simulink model "Simulator_weighted_inv"  (R2016a)
settings: Solver=ode45  StartTime=0.0  StopTime=100  RelTol=1e-3
values from neighbouring files (symbols this model uses):
  A_Servo = [0 1 0; 0 0 1 ; -B4/B1 -B3/B1 -B2/B1]    [Parameters.m]
  B_Servo = [0 ; 0 ; B0/B1]    [Parameters.m]
  C_Servo = eye(3)    [Parameters.m]
  delay_Kaltitude = 1    [Parameters.m]
  dLMN = [dLdp  0    0 ... (first row only)    [Parameters.m]
  g = 9.81    [Parameters.m]
  I_Pi = diag([8.450e-5 8.450e-5 4.580e-5])    [Parameters.m]
  In = diag([Ixx Iyy Izz])    [Parameters.m]
  InInv = In\eye(3)    [Parameters.m]
  KaD = 5.4    [Parameters.m]
  KaI = 3.6    [Parameters.m]
  KaN = 38    [Parameters.m]
  KaP = 8.0    (= 8)    [Parameters.m]
  Kba = sqrt(KaD/KaI)    [Parameters.m]
  Kbp = sqrt(Kdp/Kip)    [Parameters.m]
  Kbq = sqrt(Kdq/Kiq)    [Parameters.m]
  Kbr = sqrt(Kdr/Kir)    [Parameters.m]
  Kd_E = Kd_N    (= 0.01)    [Parameters.m]
  Kd_N = 0.01    [Parameters.m]
  Kd_u = Kd_v    (= 0.29)    [Parameters.m]
  Kd_v = 0.290    (= 0.29)    [Parameters.m]
  Kdp = 0.00534    [Parameters.m]
  Kdq = Kdp    (= 0.00534)    [Parameters.m]
  Kdr = 0.0153    [Parameters.m]
  Kinv = wpinv(K,W)    [Parameters.m]
  Kip = 0.697    [Parameters.m]
  Kiq = Kip    (= 0.697)    [Parameters.m]
  Kir = 0.125    [Parameters.m]
  Kp_E = Kp_N    (= 0.15)    [Parameters.m]
  Kp_N = 0.15    [Parameters.m]
  Kp_u = Kp_v    (= 6.3)    [Parameters.m]
  Kp_v = 6.3    [Parameters.m]
  KPD = KRD    (= 0.0584)    [Parameters.m]
  KPP = KRP    (= 1.61)    [Parameters.m]
  Kpp = 0.3    [Parameters.m]
  Kpq = Kpp    (= 0.3)    [Parameters.m]
  Kpr = 0.135    [Parameters.m]
  Kq = Cq*ro*A*R^3    (= 2.88925724261e-07)    [Parameters.m]
  KRD = 0.0584    [Parameters.m]
  KRP = 1.61    [Parameters.m]
  Kt = Ct*ro*A*R^2    (= 2.46191978476e-05)    [Parameters.m]
  m = 1.900    (= 1.9)    [Parameters.m]
  Mb = diag([m m m])    [Parameters.m]
  MbInv = Mb\eye(3)    [Parameters.m]
  N = 1/Tf    (= 100)    [Parameters.m]
  N_tras = 100    [Parameters.m]
  pitchMax = pi/6    (= 0.523598775598)    [Parameters.m]
  rollMax = pi/6    (= 0.523598775598)    [Parameters.m]
  satp = 1.5    [Parameters.m]
  satq = 1.5    [Parameters.m]
  satr = 1    [Parameters.m]
  tau = 0.055257    [Parameters.m]
  tc = 1/fc    (= 0.01)    [Parameters.m]
  x1 = [m q]    [Parameters.m]
  yawRateMax = pi/2    (= 1.57079632679)    [Parameters.m]
undefined symbols (not defined in the file or in its folder): Kp, KPI, KRI, sigbuilder_block
libraries: simulink x10, aerolibutil x10
(part 1 of 2)
settings Model: PauseTimes=2  Creator=Claudio  LastModifiedBy=Claudio
settings SolverCC: MaxConsecutiveMinStep=15
settings DataIOCC: SaveFormat=Array
settings HardwareCC: ProdBitPerPointer=32  ProdLargestAtomicFloat=None  ProdIntDivRoundTo=Undefined  ProdEndianess=Unspecified  ProdWordSize=32  ProdHWDeviceType=32-bit Generic
settings ModelReferenceCC: PropagateSignalLabelsOutOfModel=off
settings ConfigComp: CovModelRefEnable=Off

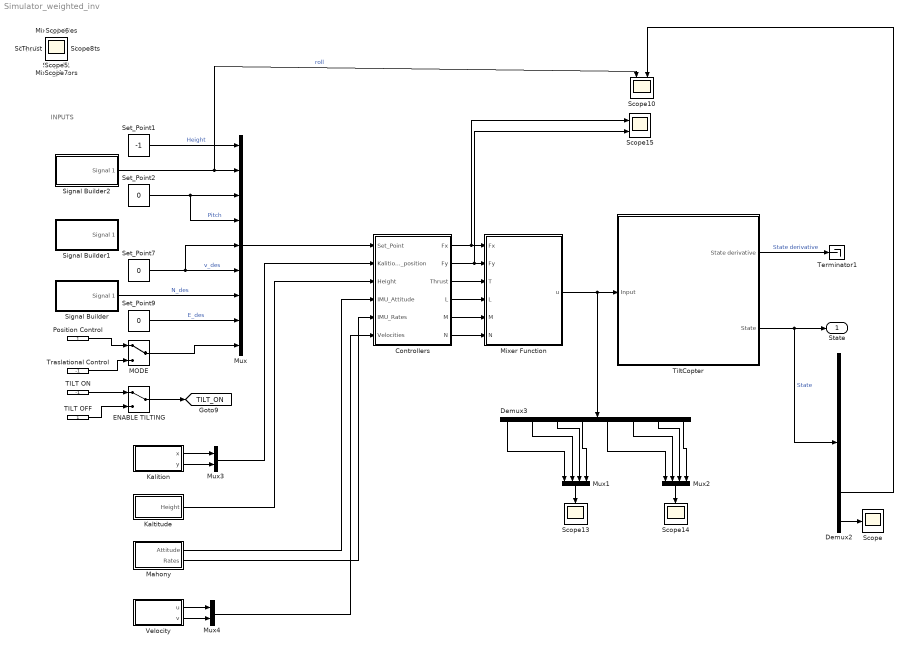
== system Simulator_weighted_inv ==
  note: INPUTS
  Controllers : Subsystem
  Demux2 : Demux  Outputs=12
  Demux3 : Demux  Outputs=8
  ENABLE TILTING : ManualSwitch
  Kalition : Subsystem
  Kaltitude : Subsystem
  MODE : ManualSwitch
  Mahony : Subsystem
  Mixer Function : Subsystem
  Mux : Mux  Inputs=9
  Mux1 : Mux
  Mux2 : Mux
  Mux3 : Mux  Inputs=2
  Mux4 : Mux  Inputs=2
  Position Control : Constant
  Scope{,1..8,11..14} (13 alike) : Scope
  Scope10 : Scope  NumInputPorts=2
  Scope15 : Scope  NumInputPorts=2
  Set_Point1 : Constant  Value=-1
  Set_Point2 : Constant  Value=0
  Set_Point7 : Constant  Value=0
  Set_Point9 : Constant  Value=0
  Signal Builder : Subsystem  Tag=STV Subsys  LoadFcn=sigbuilder_block('load');  StartFcn=sigbuilder_block('start');  StopFcn=sigbuilder_block('stop');  ClipboardFcn=sigbuilder_block('clipboard');  mask(Sigbuilder block){}
      mask help: Simulink:masks:SigbuilderBlock_MD
      mask init:
      | if ~strcmp(get_param(bdroot(gcbh),'SimulationStatus'),'stopped') tuvar = sigbuilder_block('maskInit'); end
      settings: CopyFcn=sigbuilder_block('copy');  DeleteFcn=sigbuilder_block('delete');  ModelCloseFcn=sigbuilder_block('modelClose');  PreSaveFcn=sigbuilder_block('preSave');  PauseFcn=sigbuilder_block('pause');  ContinueFcn=sigbuilder_block('continue');  NameChangeFcn=sigbuilder_block('namechange');  OpenFcn=sigbuilder_block('open',[240 98.25 550.5 359.25 ]);  CloseFcn=sigbuilder_block('close');
      mask Display: plot(0, 0, 100, 100,[2, 2, 32, 32, 2], [68, 8, 8, 68, 68],[32, 2], [38, 38], [32, 19, 2],[53, 60, 44], [32, 17, 17, 2],[16, 16, 31, 31]);txt = getActiveGroup(gcbh);text(2, 100, txt,'verticalAlignment', 'top');
  Signal Builder1 : Subsystem  Tag=STV Subsys  LoadFcn=sigbuilder_block('load');  StartFcn=sigbuilder_block('start');  StopFcn=sigbuilder_block('stop');  ClipboardFcn=sigbuilder_block('clipboard');  mask(Sigbuilder block){}
      mask help: Simulink:masks:SigbuilderBlock_MD
      mask init:
      | if ~strcmp(get_param(bdroot(gcbh),'SimulationStatus'),'stopped') tuvar = sigbuilder_block('maskInit'); end
      settings: CopyFcn=sigbuilder_block('copy');  DeleteFcn=sigbuilder_block('delete');  ModelCloseFcn=sigbuilder_block('modelClose');  PreSaveFcn=sigbuilder_block('preSave');  PauseFcn=sigbuilder_block('pause');  ContinueFcn=sigbuilder_block('continue');  NameChangeFcn=sigbuilder_block('namechange');  OpenFcn=sigbuilder_block('open',[437.25 153 550.5 359.25 ]);  CloseFcn=sigbuilder_block('close');
      mask Display: plot(0, 0, 100, 100,[2, 2, 32, 32, 2], [68, 8, 8, 68, 68],[32, 2], [38, 38], [32, 19, 2],[53, 60, 44], [32, 17, 17, 2],[16, 16, 31, 31]);txt = getActiveGroup(gcbh);text(2, 100, txt,'verticalAlignment', 'top');
  Signal Builder2 : Subsystem  Tag=STV Subsys  LoadFcn=sigbuilder_block('load');  StartFcn=sigbuilder_block('start');  StopFcn=sigbuilder_block('stop');  ClipboardFcn=sigbuilder_block('clipboard');  mask(Sigbuilder block){}
      mask help: Simulink:masks:SigbuilderBlock_MD
      mask init:
      | if ~strcmp(get_param(bdroot(gcbh),'SimulationStatus'),'stopped') tuvar = sigbuilder_block('maskInit'); end
      settings: CopyFcn=sigbuilder_block('copy');  DeleteFcn=sigbuilder_block('delete');  ModelCloseFcn=sigbuilder_block('modelClose');  PreSaveFcn=sigbuilder_block('preSave');  PauseFcn=sigbuilder_block('pause');  ContinueFcn=sigbuilder_block('continue');  NameChangeFcn=sigbuilder_block('namechange');  OpenFcn=sigbuilder_block('open',[437.25 153 550.5 359.25 ]);  CloseFcn=sigbuilder_block('close');
      mask Display: plot(0, 0, 100, 100,[2, 2, 32, 32, 2], [68, 8, 8, 68, 68],[32, 2], [38, 38], [32, 19, 2],[53, 60, 44], [32, 17, 17, 2],[16, 16, 31, 31]);txt = getActiveGroup(gcbh);text(2, 100, txt,'verticalAlignment', 'top');
  TILT OFF : Constant
  TILT ON : Constant  Value=-1
  Terminator1 : Terminator
  TiltCopter : Subsystem
      mask Display:
      | image(imread('TiltCopter_Model.png'))
      | port_label('input',1,'u')
      | port_label('output',1,'Xdot')
      | port_label('output',2,'X')
  Traslational Control : Constant  Value=-1
  Velocity : Subsystem
  State : Outport
  Forces : Scope
  Mixer_Angles : Scope
  Mixer_Motors : Scope
  Moments : Scope
  Thrust : Scope
  tag scope: TILT_ON=global
  wires:
  TiltCopter/2(State) -> Demux2/1, State/1  "State"
  TiltCopter/1(State derivative) -> Terminator1/1  "State derivative"
  Controllers/3(Thrust) -> Mixer Function/3(T)
  Controllers/4(L) -> Mixer Function/4(L)
  Controllers/5(M) -> Mixer Function/5(M)
  Set_Point1/1 -> Mux/1  "Height"
  Set_Point2/1 -> Mux/4, Mux/3  "Pitch"
  Mux/1 -> Controllers/1(Set_Point)
  Set_Point7/1 -> Mux/5, Mux/6  "v_des"
  Set_Point9/1 -> Mux/8  "E_des"
  Position Control/1 -> MODE/1
  Traslational Control/1 -> MODE/2
  MODE/1 -> Mux/9
  Mixer Function/1(u) -> Demux3/1, TiltCopter/1(Input)
  Mux1/1 -> Scope13/1
  Demux3/1 -> Mux1/1
  Demux3/2 -> Mux1/2
  Demux3/3 -> Mux1/3
  Demux3/4 -> Mux1/4
  Mux2/1 -> Scope14/1
  Demux3/5 -> Mux2/1
  Demux3/6 -> Mux2/2
  Demux3/7 -> Mux2/3
  Demux3/8 -> Mux2/4
  Kalition/2(y) -> Mux3/2
  Kalition/1(x) -> Mux3/1
  Mux3/1 -> Controllers/2(Kalition_position)
  Kaltitude/1(Height) -> Controllers/3(Height)
  Mahony/1(Attitude) -> Controllers/4(IMU_Attitude)
  Mahony/2(Rates) -> Controllers/5(IMU_Rates)
  Velocity/2(v) -> Mux4/2
  Velocity/1(u) -> Mux4/1
  Mux4/1 -> Controllers/6(Velocities)
  Controllers/1(Fx) -> Scope15/1, Mixer Function/1(Fx)
  Controllers/2(Fy) -> Scope15/2, Mixer Function/2(Fy)
  TILT ON/1 -> ENABLE TILTING/1
  TILT OFF/1 -> ENABLE TILTING/2
  ENABLE TILTING/1 -> [TILT_ON]
  Controllers/6(N) -> Mixer Function/6(N)
  Signal Builder2/1(Signal 1) -> Scope10/1, Mux/2  "roll"
  Demux2/10 -> Scope10/2
  Demux2/12 -> Scope/1
  Signal Builder/1(Signal 1) -> Mux/7  "N_des"

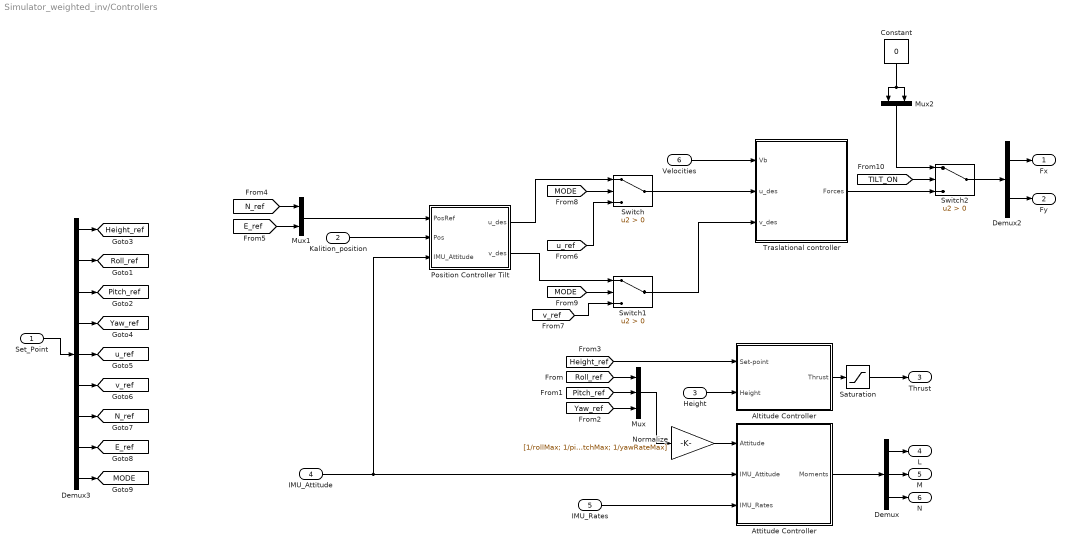
== system Simulator_weighted_inv/Controllers ==
  Set_Point : Inport
  Kalition_position : Inport  Port=2
  Height : Inport  Port=3
  IMU_Attitude : Inport  Port=4
  IMU_Rates : Inport  Port=5
  Velocities : Inport  Port=6
  Altitude Controller : Subsystem
  Attitude Controller : Subsystem
  Constant : Constant  Value=0
  Demux : Demux  Outputs=3
  Demux2 : Demux  Outputs=2
  Demux3 : Demux  Outputs=9
  Mux : Mux  Inputs=3
  Mux1 : Mux  Inputs=2
  Mux2 : Mux  Inputs=2
  Normalize : Gain  Gain=[1/rollMax; 1/pitchMax; 1/yawRateMax]
  Position Controller Tilt : Subsystem
  Saturation : Saturate  UpperLimit=0  LowerLimit=-80
  Switch : Switch  Criteria=u2 > Threshold
  Switch1 : Switch  Criteria=u2 > Threshold
  Switch2 : Switch  Criteria=u2 > Threshold
  Traslational controller : Subsystem
  Fx : Outport
  Fy : Outport  Port=2
  Thrust : Outport  Port=3
  L : Outport  Port=4
  M : Outport  Port=5
  N : Outport  Port=6
  tag scope: E_ref=global, Height_ref=global, MODE=global, N_ref=global, Pitch_ref=global, Roll_ref=global, Yaw_ref=global, u_ref=global, v_ref=global
  wires:
  IMU_Rates/1 -> Attitude Controller/3(IMU_Rates)
  Demux/1 -> L/1
  Demux/2 -> M/1
  Demux/3 -> N/1
  [Pitch_ref] -> Mux/2
  [Yaw_ref] -> Mux/3
  IMU_Attitude/1 -> Position Controller Tilt/3(IMU_Attitude), Attitude Controller/2(IMU_Attitude)
  Mux/1 -> Normalize/1
  Normalize/1 -> Attitude Controller/1(Attitude)
  [Height_ref] -> Altitude Controller/1(Set-point)
  Height/1 -> Altitude Controller/2(Height)
  Altitude Controller/1(Thrust) -> Saturation/1
  Saturation/1 -> Thrust/1
  Attitude Controller/1(Moments) -> Demux/1
  [Roll_ref] -> Mux/1
  Demux2/1 -> Fx/1
  Demux2/2 -> Fy/1
  Velocities/1 -> Traslational controller/1(Vb)
  Set_Point/1 -> Demux3/1
  Demux3/2 -> [Roll_ref]
  Demux3/1 -> [Height_ref]
  Demux3/3 -> [Pitch_ref]
  Demux3/4 -> [Yaw_ref]
  Demux3/5 -> [u_ref]
  Demux3/6 -> [v_ref]
  Demux3/7 -> [N_ref]
  Demux3/8 -> [E_ref]
  Mux1/1 -> Position Controller Tilt/1(PosRef)
  Kalition_position/1 -> Position Controller Tilt/2(Pos)
  [N_ref] -> Mux1/1
  [E_ref] -> Mux1/2
  Demux3/9 -> [MODE]
  Position Controller Tilt/1(u_des) -> Switch/1
  Position Controller Tilt/2(v_des) -> Switch1/1
  Switch/1 -> Traslational controller/2(u_des)
  [u_ref] -> Switch/3
  [v_ref] -> Switch1/3
  [MODE] -> Switch/2
  [MODE] -> Switch1/2
  Switch1/1 -> Traslational controller/3(v_des)
  Switch2/1 -> Demux2/1
  Traslational controller/1(Forces) -> Switch2/3
  Constant/1 -> Mux2/1, Mux2/2
  Mux2/1 -> Switch2/1
  [TILT_ON] -> Switch2/2

== system Simulator_weighted_inv/Kalition ==
  Demux : Demux  Outputs=3
  Terminator : Terminator
  x : Outport
  y : Outport  Port=2
  wires:
  Demux/1 -> x/1  "x"
  Demux/3 -> Terminator/1  "z"
  Demux/2 -> y/1  "y"
  [P_b] -> Demux/1

== system Simulator_weighted_inv/Kaltitude ==
  Bias_u : Bias
  Demux : Demux  Outputs=3
  Sum : Sum  Inputs=|++
  Terminator1 : Terminator
  Terminator2 : Terminator
  Transport Delay : TransportDelay  DelayTime=delay_Kaltitude*tc
  White Noise_u : RandomNumber  DisableCoverage=on  Variance=0*0.00001  SampleTime=0.01
  Zero-Order Hold : ZeroOrderHold  SampleTime=tc
  Height : Outport
  wires:
  Sum/1 -> Zero-Order Hold/1
  Demux/2 -> Terminator1/1  "E"
  [P_e] -> Demux/1
  Bias_u/1 -> Sum/1
  White Noise_u/1 -> Sum/2
  Demux/1 -> Terminator2/1  "N"
  Zero-Order Hold/1 -> Transport Delay/1
  Demux/3 -> Bias_u/1  "D"
  Transport Delay/1 -> Height/1

== system Simulator_weighted_inv/Mahony ==
  Attitude : Outport
  Rates : Outport  Port=2
  wires:
  [Omega_b] -> Rates/1
  [Alpha_e] -> Attitude/1

== system Simulator_weighted_inv/Mixer Function ==
  Fx : Inport
  Fy : Inport  Port=2
  T : Inport  Port=3
  L : Inport  Port=4
  M : Inport  Port=5
  N : Inport  Port=6
  Mux2 : Mux  Inputs=8
  To Workspace : ToWorkspace  VariableName=Uscita_quad  SaveFormat=Structure With Time  SampleTime=-1
  Weighted mixer : Subsystem
  u : Outport
  wires:
  Mux2/1 -> u/1, To Workspace/1
  Fy/1 -> Weighted mixer/2(Fy)
  Fx/1 -> Weighted mixer/1(Fx)
  T/1 -> Weighted mixer/3(T)
  M/1 -> Weighted mixer/5(M)
  Weighted mixer/4(Th4 [%]) -> Mux2/4
  Weighted mixer/3(Th3 [%]) -> Mux2/3
  Weighted mixer/2(Th2 [%]) -> Mux2/2
  Weighted mixer/1(Th1 [%]) -> Mux2/1
  Weighted mixer/5(Alpha1 [deg]) -> Mux2/5
  Weighted mixer/7(Alpha3 [deg]) -> Mux2/7
  Weighted mixer/8(Alpha4 [deg]) -> Mux2/8
  Weighted mixer/6(Alpha2 [deg]) -> Mux2/6
  L/1 -> Weighted mixer/4(L)
  N/1 -> Weighted mixer/6(N)

== system Simulator_weighted_inv/Signal Builder ==
  Demux : Demux  Tag=STV Demux  Outputs=1
  FromWs : FromWorkspace  Tag=STV FromWs  VariableName=tuvar  SampleTime=0
      SigBuilderData=|
      | common.afterFinalStr = 'Extrapolate'
      | common.sampleTime = 0
      | dataSet.timeRange = [0 40]
      | dataSet.name = 'Group 1'
      | sbobj.Groups.Name = 'Group 1'
      | sbobj.Groups.Signals.Name = 'Signal 1'
      | sbobj.Groups.Signals.XData = [0 20 23 40]
      | sbobj.Groups.Signals.YData = [0 0 0.99 1]
      | sbobj.Groups.TimeRange = [0 40]
  Signal 1 : Outport  Tag=STV Outport
  wires:
  Demux/1 -> Signal 1/1
  FromWs/1 -> Demux/1

== system Simulator_weighted_inv/Signal Builder1 ==
  Demux : Demux  Tag=STV Demux  Outputs=1
  FromWs : FromWorkspace  Tag=STV FromWs  VariableName=tuvar  SampleTime=0
      SigBuilderData=|
      | common.afterFinalStr = 'Extrapolate'
      | common.sampleTime = 0
      | dataSet.timeRange = [0 10]
      | dataSet.name = 'Group 1'
      | sbobj.Groups.Name = 'Group 1'
      | sbobj.Groups.Signals.Name = 'Signal 1'
      | sbobj.Groups.Signals.XData = [0 2 3 4 5 6 10]
      | sbobj.Groups.Signals.YData = [0 -0.001 0.5 0.5 0 0 0]
  Signal 1 : Outport  Tag=STV Outport
  wires:
  FromWs/1 -> Demux/1
  Demux/1 -> Signal 1/1

== system Simulator_weighted_inv/Signal Builder2 ==
  Demux : Demux  Tag=STV Demux  Outputs=1
  FromWs : FromWorkspace  Tag=STV FromWs  VariableName=tuvar  SampleTime=0
      SigBuilderData=|
      | common.afterFinalStr = 'Extrapolate'
      | common.sampleTime = 0
      | dataSet.timeRange = [0 10]
      | dataSet.name = 'Group 1'
      | sbobj.Groups.Name = 'Group 1'
      | sbobj.Groups.Signals.Name = 'Signal 1'
      | sbobj.Groups.Signals.XData = [0 3 5 7 8.58 10]
      | sbobj.Groups.Signals.YData = [0 0 0.17 0.17 0 0]
  Signal 1 : Outport  Tag=STV Outport
  wires:
  Demux/1 -> Signal 1/1
  FromWs/1 -> Demux/1

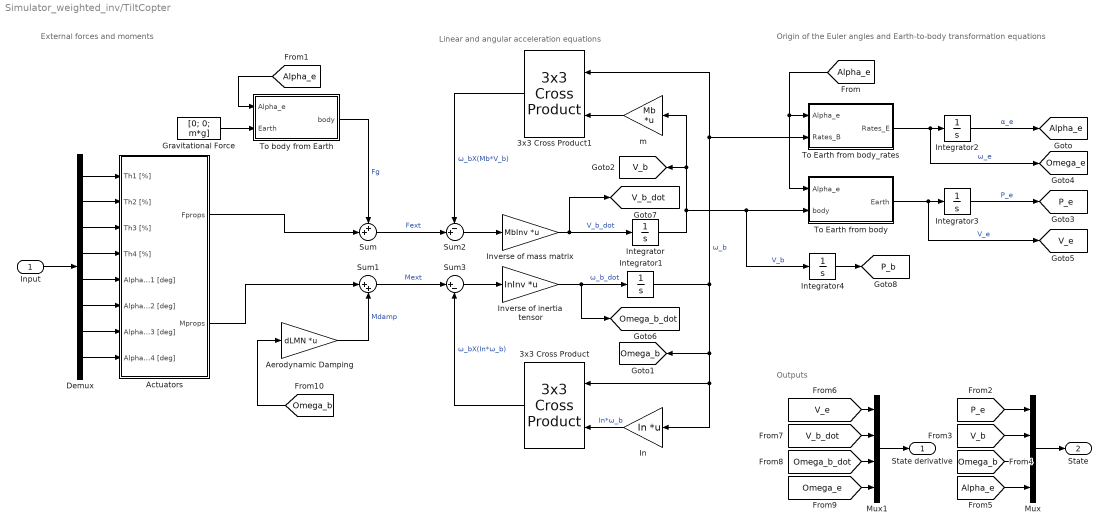
== system Simulator_weighted_inv/TiltCopter ==
  note: External forces and moments
  note: Outputs
  note: Origin of the Euler angles and Earth-to-body transformation equations
  note: Linear and angular acceleration equations
  Input : Inport
  3x3 Cross Product : aerolibutil/3x3 Cross Product
  3x3 Cross Product1 : aerolibutil/3x3 Cross Product
  Actuators : Subsystem
  Aerodynamic Damping : Gain  Gain=dLMN  Multiplication=Matrix(K*u)
  Demux : Demux  Outputs=8
  Gravitational Force : Constant  Value=[0; 0; m*g]
  In : Gain  Gain=In  Multiplication=Matrix(K*u)
  Integrator : Integrator  InitialCondition=[0; 0; 0]  UpperSaturationLimit=20
  Integrator{1..4} (4 alike) : Integrator  InitialCondition=[0; 0; 0]
  Inverse of inertia tensor : Gain  Gain=InInv  Multiplication=Matrix(K*u)
  Inverse of mass matrix : Gain  Gain=MbInv  Multiplication=Matrix(K*u)
  Mux : Mux
  Mux1 : Mux
  Sum : Sum  Inputs=++|
  Sum1 : Sum  Inputs=|++
  Sum2 : Sum  Inputs=-+|
  Sum3 : Sum  Inputs=|+-
  To Earth from body : MATLAB Function  TreatAsAtomicUnit=on
  To Earth from body_rates : MATLAB Function  TreatAsAtomicUnit=on
  To body from Earth : MATLAB Function  TreatAsAtomicUnit=on
  m : Gain  Gain=Mb  Multiplication=Matrix(K*u)
  State derivative : Outport
  State : Outport  Port=2
  tag scope: Alpha_e=global, Omega_b=global, Omega_b_dot=global, Omega_e=global, P_b=global, P_e=global, V_b=global, V_b_dot=global, V_e=global
  wires:
  To Earth from body_rates/1(Rates_E) -> Integrator2/1, [Omega_e]  "ω_e"
  [P_e] -> Mux/1
  3x3 Cross Product/1 -> Sum3/2  "ω_bX(In*ω_b)"
  [V_b_dot] -> Mux1/2
  Mux/1 -> State/1
  Mux1/1 -> State derivative/1
  [V_b] -> Mux/2
  [Alpha_e] -> Mux/4
  [Omega_b] -> Mux/3
  Demux/4 -> Actuators/4(Th4 [%])
  [Omega_e] -> Mux1/4
  [Omega_b_dot] -> Mux1/3
  [V_e] -> Mux1/1
  Demux/3 -> Actuators/3(Th3 [%])
  Inverse of mass matrix/1 -> Integrator/1, [V_b_dot]  "V_b_dot"
  Integrator/1 -> Integrator4/1, To Earth from body/2(body), m/1, [V_b]  "V_b"
  [Alpha_e] -> To Earth from body/1(Alpha_e), To Earth from body_rates/1(Alpha_e)
  Integrator1/1 -> To Earth from body_rates/2(Rates_B), 3x3 Cross Product1/1, 3x3 Cross Product/1, In/1, [Omega_b]  "ω_b"
  Sum3/1 -> Inverse of inertia tensor/1
  Sum2/1 -> Inverse of mass matrix/1
  m/1 -> 3x3 Cross Product1/2
  Sum/1 -> Sum2/2  "Fext"
  Sum1/1 -> Sum3/1  "Mext"
  Demux/1 -> Actuators/1(Th1 [%])
  Demux/2 -> Actuators/2(Th2 [%])
  Inverse of inertia tensor/1 -> Integrator1/1, [Omega_b_dot]  "ω_b_dot"
  3x3 Cross Product1/1 -> Sum2/1  "ω_bX(Mb*V_b)"
  Integrator2/1 -> [Alpha_e]  "α_e"
  Aerodynamic Damping/1 -> Sum1/2  "Mdamp"
  Integrator3/1 -> [P_e]  "P_e"
  In/1 -> 3x3 Cross Product/2  "In*ω_b"
  [Omega_b] -> Aerodynamic Damping/1
  To Earth from body/1(Earth) -> [V_e], Integrator3/1  "V_e"
  To body from Earth/1(body) -> Sum/1  "Fg"
  Gravitational Force/1 -> To body from Earth/2(Earth)
  [Alpha_e] -> To body from Earth/1(Alpha_e)
  Input/1 -> Demux/1
  Demux/5 -> Actuators/5(Alpha_1 [deg])
  Demux/6 -> Actuators/6(Alpha_2 [deg])
  Demux/7 -> Actuators/7(Alpha_3 [deg])
  Demux/8 -> Actuators/8(Alpha_4 [deg])
  Actuators/1(Fprops) -> Sum/2
  Actuators/2(Mprops) -> Sum1/1
  Integrator4/1 -> [P_b]

== system Simulator_weighted_inv/Velocity ==
  Demux : Demux  Outputs=3
  Terminator : Terminator
  u : Outport
  v : Outport  Port=2
  wires:
  Demux/2 -> v/1  "v"
  [V_b] -> Demux/1
  Demux/3 -> Terminator/1  "w"
  Demux/1 -> u/1  "u"

== system Simulator_weighted_inv/Controllers/Altitude Controller ==
  Set-point : Inport
  Height : Inport  Port=2
  Constant : Constant  Value=m*g
  Normalize : Gain
  PD Controller : simulink/Continuous/PID Controller  Controller=PID  TimeDomain=Continuous-time  SampleTime=-1  IntegratorMethod=Forward Euler  FilterMethod=Trapezoidal  Form=Parallel  UseFilter=on  ControllerParametersSource=internal  P=KaP  I=KaI  D=KaD  N=KaN  InitialConditionSource=internal  InitialConditionForIntegrator=0  InitialConditionForFilter=0  ExternalReset=none  LimitOutput=on  UpperSaturationLimit=10  LowerSaturationLimit=-10  LinearizeAsGain=on  AntiWindupMode=back-calculation  Kb=Kba  TrackingMode=off  Kt=1  PParamMin=[]  PParamMax=[]  IParamMin=[]  IParamMax=[]  DParamMin=[]  DParamMax=[]  NParamMin=[]  NParamMax=[]  KbParamMin=[]  KbParamMax=[]  KtParamMin=[]  KtParamMax=[]  POutMin=[]  POutMax=[]  IOutMin=[]  IOutMax=[]  DOutMin=[]  DOutMax=[]  NOutMin=[]  NOutMax=[]  KbOutMin=[]  KbOutMax=[]  KtOutMin=[]  KtOutMax=[]  IntegratorOutMin=[]  IntegratorOutMax=[]  FilterOutMin=[]  FilterOutMax=[]  SumOutMin=[]  SumOutMax=[]  SumI1OutMin=[]  SumI1OutMax=[]  SumI2OutMin=[]  SumI2OutMax=[]  SumI3OutMin=[]  SumI3OutMax=[]  SumDOutMin=[]  SumDOutMax=[]  SaturationOutMin=[]  SaturationOutMax=[]  IntegratorContinuousStateAttributes=''  IntegratorStateMustResolveToSignalObject=off  IntegratorRTWStateStorageClass=Auto  FilterContinuousStateAttributes=''  FilterStateMustResolveToSignalObject=off  FilterRTWStateStorageClass=Auto  DifferentiatorICPrevScaledInput=0  DifferentiatorOutMin=[]  DifferentiatorOutMax=[]
  Sum1 : Sum  Inputs=-+|
  Sum2 : Sum  Inputs=|+-
  Thrust : Outport
  wires:
  Sum2/1 -> PD Controller/1
  Height/1 -> Sum2/2
  Sum1/1 -> Thrust/1
  Constant/1 -> Sum1/1
  Set-point/1 -> Sum2/1
  PD Controller/1 -> Normalize/1
  Normalize/1 -> Sum1/2

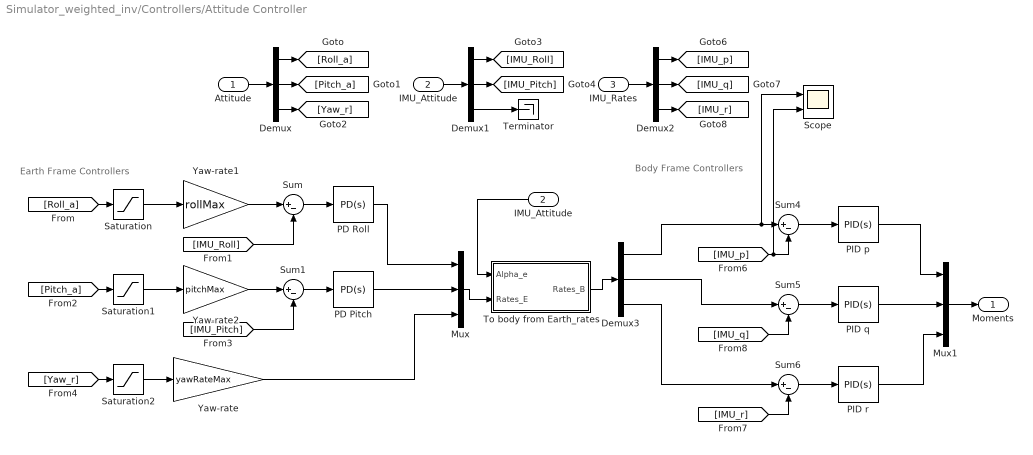
== system Simulator_weighted_inv/Controllers/Attitude Controller ==
  note: Body Frame Controllers
  note: Earth Frame Controllers
  Attitude : Inport
  IMU_Attitude : Inport  Port=2
  IMU_Rates : Inport  Port=3
  Demux{,1..3} (4 alike) : Demux  Outputs=3
  "IMU_Attitude " : InportShadow  Port=2
  Mux : Mux  Inputs=3
  Mux1 : Mux  Inputs=3
  PD Pitch : simulink/Continuous/PID Controller  Controller=PD  TimeDomain=Continuous-time  SampleTime=-1  IntegratorMethod=Forward Euler  FilterMethod=Forward Euler  Form=Parallel  UseFilter=on  ControllerParametersSource=internal  P=KPP  I=KPI  D=KPD  N=N  InitialConditionSource=internal  InitialConditionForIntegrator=0  InitialConditionForFilter=0  ExternalReset=none  LimitOutput=off  UpperSaturationLimit=inf  LowerSaturationLimit=-inf  LinearizeAsGain=on  AntiWindupMode=none  Kb=1  TrackingMode=off  Kt=1  PParamMin=[]  PParamMax=[]  IParamMin=[]  IParamMax=[]  DParamMin=[]  DParamMax=[]  NParamMin=[]  NParamMax=[]  KbParamMin=[]  KbParamMax=[]  KtParamMin=[]  KtParamMax=[]  POutMin=[]  POutMax=[]  IOutMin=[]  IOutMax=[]  DOutMin=[]  DOutMax=[]  NOutMin=[]  NOutMax=[]  KbOutMin=[]  KbOutMax=[]  KtOutMin=[]  KtOutMax=[]  IntegratorOutMin=[]  IntegratorOutMax=[]  FilterOutMin=[]  FilterOutMax=[]  SumOutMin=[]  SumOutMax=[]  SumI1OutMin=[]  SumI1OutMax=[]  SumI2OutMin=[]  SumI2OutMax=[]  SumI3OutMin=[]  SumI3OutMax=[]  SumDOutMin=[]  SumDOutMax=[]  SaturationOutMin=[]  SaturationOutMax=[]  IntegratorContinuousStateAttributes=''  IntegratorStateMustResolveToSignalObject=off  IntegratorRTWStateStorageClass=Auto  FilterContinuousStateAttributes=''  FilterStateMustResolveToSignalObject=off  FilterRTWStateStorageClass=Auto  DifferentiatorICPrevScaledInput=0  DifferentiatorOutMin=[]  DifferentiatorOutMax=[]
  PD Roll : simulink/Continuous/PID Controller  Controller=PD  TimeDomain=Continuous-time  SampleTime=-1  IntegratorMethod=Forward Euler  FilterMethod=Forward Euler  Form=Parallel  UseFilter=on  ControllerParametersSource=internal  P=KRP  I=KRI  D=KRD  N=N  InitialConditionSource=internal  InitialConditionForIntegrator=0  InitialConditionForFilter=0  ExternalReset=none  LimitOutput=off  UpperSaturationLimit=inf  LowerSaturationLimit=-inf  LinearizeAsGain=on  AntiWindupMode=none  Kb=1  TrackingMode=off  Kt=1  PParamMin=[]  PParamMax=[]  IParamMin=[]  IParamMax=[]  DParamMin=[]  DParamMax=[]  NParamMin=[]  NParamMax=[]  KbParamMin=[]  KbParamMax=[]  KtParamMin=[]  KtParamMax=[]  POutMin=[]  POutMax=[]  IOutMin=[]  IOutMax=[]  DOutMin=[]  DOutMax=[]  NOutMin=[]  NOutMax=[]  KbOutMin=[]  KbOutMax=[]  KtOutMin=[]  KtOutMax=[]  IntegratorOutMin=[]  IntegratorOutMax=[]  FilterOutMin=[]  FilterOutMax=[]  SumOutMin=[]  SumOutMax=[]  SumI1OutMin=[]  SumI1OutMax=[]  SumI2OutMin=[]  SumI2OutMax=[]  SumI3OutMin=[]  SumI3OutMax=[]  SumDOutMin=[]  SumDOutMax=[]  SaturationOutMin=[]  SaturationOutMax=[]  IntegratorContinuousStateAttributes=''  IntegratorStateMustResolveToSignalObject=off  IntegratorRTWStateStorageClass=Auto  FilterContinuousStateAttributes=''  FilterStateMustResolveToSignalObject=off  FilterRTWStateStorageClass=Auto  DifferentiatorICPrevScaledInput=0  DifferentiatorOutMin=[]  DifferentiatorOutMax=[]
  PID p : simulink/Continuous/PID Controller  Controller=PID  TimeDomain=Continuous-time  SampleTime=-1  IntegratorMethod=Forward Euler  FilterMethod=Forward Euler  Form=Parallel  UseFilter=on  ControllerParametersSource=internal  P=Kpp  I=Kip  D=Kdp  N=N  InitialConditionSource=internal  InitialConditionForIntegrator=0  InitialConditionForFilter=0  ExternalReset=none  LimitOutput=on  UpperSaturationLimit=satp  LowerSaturationLimit=-satp  LinearizeAsGain=on  AntiWindupMode=back-calculation  Kb=Kbp  TrackingMode=off  Kt=1  PParamMin=[]  PParamMax=[]  IParamMin=[]  IParamMax=[]  DParamMin=[]  DParamMax=[]  NParamMin=[]  NParamMax=[]  KbParamMin=[]  KbParamMax=[]  KtParamMin=[]  KtParamMax=[]  POutMin=[]  POutMax=[]  IOutMin=[]  IOutMax=[]  DOutMin=[]  DOutMax=[]  NOutMin=[]  NOutMax=[]  KbOutMin=[]  KbOutMax=[]  KtOutMin=[]  KtOutMax=[]  IntegratorOutMin=[]  IntegratorOutMax=[]  FilterOutMin=[]  FilterOutMax=[]  SumOutMin=[]  SumOutMax=[]  SumI1OutMin=[]  SumI1OutMax=[]  SumI2OutMin=[]  SumI2OutMax=[]  SumI3OutMin=[]  SumI3OutMax=[]  SumDOutMin=[]  SumDOutMax=[]  SaturationOutMin=[]  SaturationOutMax=[]  IntegratorContinuousStateAttributes=''  IntegratorStateMustResolveToSignalObject=off  IntegratorRTWStateStorageClass=Auto  FilterContinuousStateAttributes=''  FilterStateMustResolveToSignalObject=off  FilterRTWStateStorageClass=Auto  DifferentiatorICPrevScaledInput=0  DifferentiatorOutMin=[]  DifferentiatorOutMax=[]
  PID q : simulink/Continuous/PID Controller  Controller=PID  TimeDomain=Continuous-time  SampleTime=-1  IntegratorMethod=Forward Euler  FilterMethod=Forward Euler  Form=Parallel  UseFilter=on  ControllerParametersSource=internal  P=Kpq  I=Kiq  D=Kdq  N=N  InitialConditionSource=internal  InitialConditionForIntegrator=0  InitialConditionForFilter=0  ExternalReset=none  LimitOutput=on  UpperSaturationLimit=satq  LowerSaturationLimit=-satq  LinearizeAsGain=on  AntiWindupMode=back-calculation  Kb=Kbq  TrackingMode=off  Kt=1  PParamMin=[]  PParamMax=[]  IParamMin=[]  IParamMax=[]  DParamMin=[]  DParamMax=[]  NParamMin=[]  NParamMax=[]  KbParamMin=[]  KbParamMax=[]  KtParamMin=[]  KtParamMax=[]  POutMin=[]  POutMax=[]  IOutMin=[]  IOutMax=[]  DOutMin=[]  DOutMax=[]  NOutMin=[]  NOutMax=[]  KbOutMin=[]  KbOutMax=[]  KtOutMin=[]  KtOutMax=[]  IntegratorOutMin=[]  IntegratorOutMax=[]  FilterOutMin=[]  FilterOutMax=[]  SumOutMin=[]  SumOutMax=[]  SumI1OutMin=[]  SumI1OutMax=[]  SumI2OutMin=[]  SumI2OutMax=[]  SumI3OutMin=[]  SumI3OutMax=[]  SumDOutMin=[]  SumDOutMax=[]  SaturationOutMin=[]  SaturationOutMax=[]  IntegratorContinuousStateAttributes=''  IntegratorStateMustResolveToSignalObject=off  IntegratorRTWStateStorageClass=Auto  FilterContinuousStateAttributes=''  FilterStateMustResolveToSignalObject=off  FilterRTWStateStorageClass=Auto  DifferentiatorICPrevScaledInput=0  DifferentiatorOutMin=[]  DifferentiatorOutMax=[]
  PID r : simulink/Continuous/PID Controller  Controller=PID  TimeDomain=Continuous-time  SampleTime=-1  IntegratorMethod=Forward Euler  FilterMethod=Forward Euler  Form=Parallel  UseFilter=on  ControllerParametersSource=internal  P=Kpr  I=Kir  D=Kdr  N=N  InitialConditionSource=internal  InitialConditionForIntegrator=0  InitialConditionForFilter=0  ExternalReset=none  LimitOutput=on  UpperSaturationLimit=satr  LowerSaturationLimit=-satr  LinearizeAsGain=on  AntiWindupMode=back-calculation  Kb=Kbr  TrackingMode=off  Kt=1  PParamMin=[]  PParamMax=[]  IParamMin=[]  IParamMax=[]  DParamMin=[]  DParamMax=[]  NParamMin=[]  NParamMax=[]  KbParamMin=[]  KbParamMax=[]  KtParamMin=[]  KtParamMax=[]  POutMin=[]  POutMax=[]  IOutMin=[]  IOutMax=[]  DOutMin=[]  DOutMax=[]  NOutMin=[]  NOutMax=[]  KbOutMin=[]  KbOutMax=[]  KtOutMin=[]  KtOutMax=[]  IntegratorOutMin=[]  IntegratorOutMax=[]  FilterOutMin=[]  FilterOutMax=[]  SumOutMin=[]  SumOutMax=[]  SumI1OutMin=[]  SumI1OutMax=[]  SumI2OutMin=[]  SumI2OutMax=[]  SumI3OutMin=[]  SumI3OutMax=[]  SumDOutMin=[]  SumDOutMax=[]  SaturationOutMin=[]  SaturationOutMax=[]  IntegratorContinuousStateAttributes=''  IntegratorStateMustResolveToSignalObject=off  IntegratorRTWStateStorageClass=Auto  FilterContinuousStateAttributes=''  FilterStateMustResolveToSignalObject=off  FilterRTWStateStorageClass=Auto  DifferentiatorICPrevScaledInput=0  DifferentiatorOutMin=[]  DifferentiatorOutMax=[]
  Saturation : Saturate  UpperLimit=1  LowerLimit=-1
  Saturation1 : Saturate  UpperLimit=1  LowerLimit=-1
  Saturation2 : Saturate  UpperLimit=1  LowerLimit=-1
  Scope : Scope  NumInputPorts=2
  Sum{,1,4..6} (5 alike) : Sum  Inputs=|+-
  Terminator : Terminator
  To body from Earth_rates : MATLAB Function  TreatAsAtomicUnit=on
  Yaw-rate : Gain  Gain=yawRateMax
  Yaw-rate1 : Gain  Gain=rollMax
  Yaw-rate2 : Gain  Gain=pitchMax
  Moments : Outport
  wires:
  Sum4/1 -> PID p/1
  IMU_Attitude/1 -> Demux1/1
  Attitude/1 -> Demux/1
  Demux/3 -> [Yaw_r]
  IMU_Rates/1 -> Demux2/1
  [IMU_Pitch] -> Sum1/2
  [Pitch_a] -> Saturation1/1
  [IMU_Roll] -> Sum/2
  [Roll_a] -> Saturation/1
  Mux1/1 -> Moments/1
  PD Roll/1 -> Mux/1
  [Yaw_r] -> Saturation2/1
  PD Pitch/1 -> Mux/2
  Sum5/1 -> PID q/1
  PID r/1 -> Mux1/3
  PID p/1 -> Mux1/1
  Sum6/1 -> PID r/1
  PID q/1 -> Mux1/2
  Demux/2 -> [Pitch_a]
  Demux2/3 -> [IMU_r]
  Demux1/1 -> [IMU_Roll]
  Demux/1 -> [Roll_a]
  Demux2/1 -> [IMU_p]
  Demux1/3 -> Terminator/1
  Demux2/2 -> [IMU_q]
  Demux1/2 -> [IMU_Pitch]
  Sum/1 -> PD Roll/1
  Sum1/1 -> PD Pitch/1
  Saturation1/1 -> Yaw-rate2/1
  Yaw-rate1/1 -> Sum/1
  Yaw-rate2/1 -> Sum1/1
  [IMU_p] -> Sum4/2, Scope/2
  Demux3/2 -> Sum5/1
  Demux3/3 -> Sum6/1
  [IMU_q] -> Sum5/2
  [IMU_r] -> Sum6/2
  Yaw-rate/1 -> Mux/3
  Saturation/1 -> Yaw-rate1/1
  Saturation2/1 -> Yaw-rate/1
  "IMU_Attitude "/1 -> To body from Earth_rates/1(Alpha_e)
  Mux/1 -> To body from Earth_rates/2(Rates_E)
  To body from Earth_rates/1(Rates_B) -> Demux3/1
  Demux3/1 -> Scope/1, Sum4/1

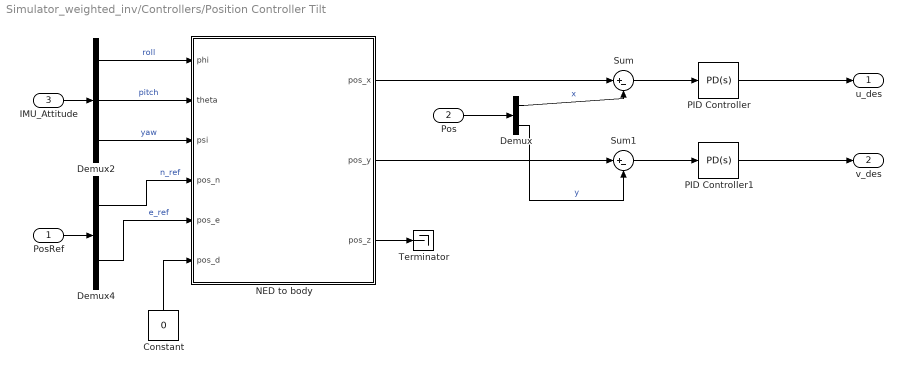
== system Simulator_weighted_inv/Controllers/Position Controller Tilt ==
  PosRef : Inport
  Pos : Inport  Port=2
  IMU_Attitude : Inport  Port=3
  Constant : Constant  Value=0
  Demux : Demux  Outputs=2
  Demux2 : Demux  Outputs=3
  Demux4 : Demux  Outputs=2
  NED to body : MATLAB Function  TreatAsAtomicUnit=on
  PID Controller : simulink/Continuous/PID Controller  Controller=PD  TimeDomain=Continuous-time  SampleTime=-1  IntegratorMethod=Forward Euler  FilterMethod=Forward Euler  Form=Parallel  UseFilter=on  ControllerParametersSource=internal  P=Kp_N  I=1  D=Kd_N  N=100  InitialConditionSource=internal  InitialConditionForIntegrator=0  InitialConditionForFilter=0  ExternalReset=none  LimitOutput=off  UpperSaturationLimit=inf  LowerSaturationLimit=-inf  LinearizeAsGain=on  AntiWindupMode=none  Kb=1  TrackingMode=off  Kt=1  PParamMin=[]  PParamMax=[]  IParamMin=[]  IParamMax=[]  DParamMin=[]  DParamMax=[]  NParamMin=[]  NParamMax=[]  KbParamMin=[]  KbParamMax=[]  KtParamMin=[]  KtParamMax=[]  POutMin=[]  POutMax=[]  IOutMin=[]  IOutMax=[]  DOutMin=[]  DOutMax=[]  NOutMin=[]  NOutMax=[]  KbOutMin=[]  KbOutMax=[]  KtOutMin=[]  KtOutMax=[]  IntegratorOutMin=[]  IntegratorOutMax=[]  FilterOutMin=[]  FilterOutMax=[]  SumOutMin=[]  SumOutMax=[]  SumI1OutMin=[]  SumI1OutMax=[]  SumI2OutMin=[]  SumI2OutMax=[]  SumI3OutMin=[]  SumI3OutMax=[]  SumDOutMin=[]  SumDOutMax=[]  SaturationOutMin=[]  SaturationOutMax=[]  IntegratorContinuousStateAttributes=''  IntegratorStateMustResolveToSignalObject=off  IntegratorRTWStateStorageClass=Auto  FilterContinuousStateAttributes=''  FilterStateMustResolveToSignalObject=off  FilterRTWStateStorageClass=Auto  DifferentiatorICPrevScaledInput=0  DifferentiatorOutMin=[]  DifferentiatorOutMax=[]
  PID Controller1 : simulink/Continuous/PID Controller  Controller=PD  TimeDomain=Continuous-time  SampleTime=-1  IntegratorMethod=Forward Euler  FilterMethod=Forward Euler  Form=Parallel  UseFilter=on  ControllerParametersSource=internal  P=Kp_E  I=1  D=Kd_E  N=100  InitialConditionSource=internal  InitialConditionForIntegrator=0  InitialConditionForFilter=0  ExternalReset=none  LimitOutput=off  UpperSaturationLimit=inf  LowerSaturationLimit=-inf  LinearizeAsGain=on  AntiWindupMode=none  Kb=1  TrackingMode=off  Kt=1  PParamMin=[]  PParamMax=[]  IParamMin=[]  IParamMax=[]  DParamMin=[]  DParamMax=[]  NParamMin=[]  NParamMax=[]  KbParamMin=[]  KbParamMax=[]  KtParamMin=[]  KtParamMax=[]  POutMin=[]  POutMax=[]  IOutMin=[]  IOutMax=[]  DOutMin=[]  DOutMax=[]  NOutMin=[]  NOutMax=[]  KbOutMin=[]  KbOutMax=[]  KtOutMin=[]  KtOutMax=[]  IntegratorOutMin=[]  IntegratorOutMax=[]  FilterOutMin=[]  FilterOutMax=[]  SumOutMin=[]  SumOutMax=[]  SumI1OutMin=[]  SumI1OutMax=[]  SumI2OutMin=[]  SumI2OutMax=[]  SumI3OutMin=[]  SumI3OutMax=[]  SumDOutMin=[]  SumDOutMax=[]  SaturationOutMin=[]  SaturationOutMax=[]  IntegratorContinuousStateAttributes=''  IntegratorStateMustResolveToSignalObject=off  IntegratorRTWStateStorageClass=Auto  FilterContinuousStateAttributes=''  FilterStateMustResolveToSignalObject=off  FilterRTWStateStorageClass=Auto  DifferentiatorICPrevScaledInput=0  DifferentiatorOutMin=[]  DifferentiatorOutMax=[]
  Sum : Sum  Inputs=|+-
  Sum1 : Sum  Inputs=|+-
  Terminator : Terminator
  u_des : Outport
  v_des : Outport  Port=2
  wires:
  Demux4/1 -> NED to body/4(pos_n)  "n_ref"
  Demux4/2 -> NED to body/5(pos_e)  "e_ref"
  PosRef/1 -> Demux4/1
  NED to body/3(pos_z) -> Terminator/1
  IMU_Attitude/1 -> Demux2/1
  Demux2/2 -> NED to body/2(theta)  "pitch"
  Constant/1 -> NED to body/6(pos_d)
  Pos/1 -> Demux/1
  Demux2/3 -> NED to body/3(psi)  "yaw"
  Demux2/1 -> NED to body/1(phi)  "roll"
  Sum/1 -> PID Controller/1
  NED to body/1(pos_x) -> Sum/1
  Demux/1 -> Sum/2  "x"
  PID Controller/1 -> u_des/1
  Sum1/1 -> PID Controller1/1
  NED to body/2(pos_y) -> Sum1/1
  Demux/2 -> Sum1/2  "y"
  PID Controller1/1 -> v_des/1

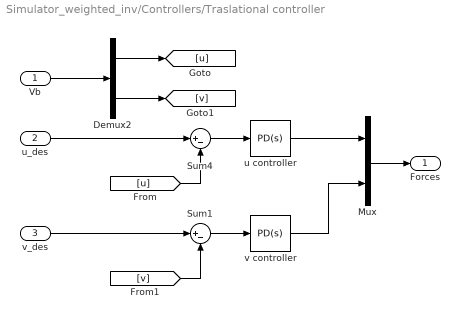
== system Simulator_weighted_inv/Controllers/Traslational controller ==
  Vb : Inport
  u_des : Inport  Port=2
  v_des : Inport  Port=3
  Demux2 : Demux  Outputs=2
  Mux : Mux  Inputs=2
  Sum1 : Sum  Inputs=|+-
  Sum4 : Sum  Inputs=|+-
  u controller : simulink/Continuous/PID Controller  Controller=PD  TimeDomain=Continuous-time  SampleTime=-1  IntegratorMethod=Forward Euler  FilterMethod=Forward Euler  Form=Parallel  UseFilter=on  ControllerParametersSource=internal  P=Kp_u  I=6  D=Kd_u  N=N_tras  InitialConditionSource=internal  InitialConditionForIntegrator=0  InitialConditionForFilter=0  ExternalReset=none  LimitOutput=off  UpperSaturationLimit=inf  LowerSaturationLimit=-inf  LinearizeAsGain=on  AntiWindupMode=none  Kb=1  TrackingMode=off  Kt=1  PParamMin=[]  PParamMax=[]  IParamMin=[]  IParamMax=[]  DParamMin=[]  DParamMax=[]  NParamMin=[]  NParamMax=[]  KbParamMin=[]  KbParamMax=[]  KtParamMin=[]  KtParamMax=[]  POutMin=[]  POutMax=[]  IOutMin=[]  IOutMax=[]  DOutMin=[]  DOutMax=[]  NOutMin=[]  NOutMax=[]  KbOutMin=[]  KbOutMax=[]  KtOutMin=[]  KtOutMax=[]  IntegratorOutMin=[]  IntegratorOutMax=[]  FilterOutMin=[]  FilterOutMax=[]  SumOutMin=[]  SumOutMax=[]  SumI1OutMin=[]  SumI1OutMax=[]  SumI2OutMin=[]  SumI2OutMax=[]  SumI3OutMin=[]  SumI3OutMax=[]  SumDOutMin=[]  SumDOutMax=[]  SaturationOutMin=[]  SaturationOutMax=[]  IntegratorContinuousStateAttributes=''  IntegratorStateMustResolveToSignalObject=off  IntegratorRTWStateStorageClass=Auto  FilterContinuousStateAttributes=''  FilterStateMustResolveToSignalObject=off  FilterRTWStateStorageClass=Auto  DifferentiatorICPrevScaledInput=0  DifferentiatorOutMin=[]  DifferentiatorOutMax=[]
  v controller : simulink/Continuous/PID Controller  Controller=PD  TimeDomain=Continuous-time  SampleTime=-1  IntegratorMethod=Forward Euler  FilterMethod=Forward Euler  Form=Parallel  UseFilter=on  ControllerParametersSource=internal  P=Kp_v  I=Kp  D=Kd_v  N=N_tras  InitialConditionSource=internal  InitialConditionForIntegrator=0  InitialConditionForFilter=0  ExternalReset=none  LimitOutput=off  UpperSaturationLimit=inf  LowerSaturationLimit=-inf  LinearizeAsGain=on  AntiWindupMode=none  Kb=1  TrackingMode=off  Kt=1  PParamMin=[]  PParamMax=[]  IParamMin=[]  IParamMax=[]  DParamMin=[]  DParamMax=[]  NParamMin=[]  NParamMax=[]  KbParamMin=[]  KbParamMax=[]  KtParamMin=[]  KtParamMax=[]  POutMin=[]  POutMax=[]  IOutMin=[]  IOutMax=[]  DOutMin=[]  DOutMax=[]  NOutMin=[]  NOutMax=[]  KbOutMin=[]  KbOutMax=[]  KtOutMin=[]  KtOutMax=[]  IntegratorOutMin=[]  IntegratorOutMax=[]  FilterOutMin=[]  FilterOutMax=[]  SumOutMin=[]  SumOutMax=[]  SumI1OutMin=[]  SumI1OutMax=[]  SumI2OutMin=[]  SumI2OutMax=[]  SumI3OutMin=[]  SumI3OutMax=[]  SumDOutMin=[]  SumDOutMax=[]  SaturationOutMin=[]  SaturationOutMax=[]  IntegratorContinuousStateAttributes=''  IntegratorStateMustResolveToSignalObject=off  IntegratorRTWStateStorageClass=Auto  FilterContinuousStateAttributes=''  FilterStateMustResolveToSignalObject=off  FilterRTWStateStorageClass=Auto  DifferentiatorICPrevScaledInput=0  DifferentiatorOutMin=[]  DifferentiatorOutMax=[]
  Forces : Outport
  wires:
  Sum4/1 -> u controller/1
  [u] -> Sum4/2
  Vb/1 -> Demux2/1
  Demux2/2 -> [v]
  Demux2/1 -> [u]
  u controller/1 -> Mux/1
  Sum1/1 -> v controller/1
  [v] -> Sum1/2
  Mux/1 -> Forces/1
  v controller/1 -> Mux/2
  u_des/1 -> Sum4/1
  v_des/1 -> Sum1/1

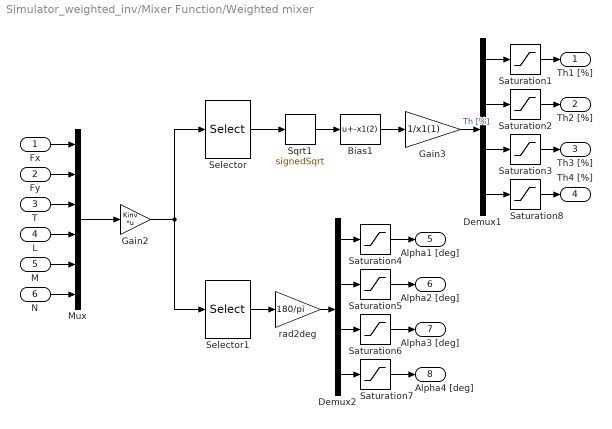
== system Simulator_weighted_inv/Mixer Function/Weighted mixer ==
  Fx : Inport
  Fy : Inport  Port=2
  T : Inport  Port=3
  L : Inport  Port=4
  M : Inport  Port=5
  N : Inport  Port=6
  Bias1 : Bias  Bias=-x1(2)
  Demux1 : Demux
  Demux2 : Demux
  Gain2 : Gain  Gain=Kinv  Multiplication=Matrix(K*u)
  Gain3 : Gain  Gain=1/x1(1)
  Mux : Mux  Inputs=6
  Saturation{1..3,8} (4 alike) : Saturate  UpperLimit=100  LowerLimit=0
  Saturation{4..7} (4 alike) : Saturate  UpperLimit=45  LowerLimit=-45
  Selector : Selector  InputPortWidth=8  IndexOptions=Index vector (dialog)  Indices=[1 2 3 4]  OutputSizes=1
  Selector1 : Selector  InputPortWidth=8  IndexOptions=Index vector (dialog)  Indices=[5 6 7 8]  OutputSizes=1
  Sqrt1 : Sqrt  Operator=signedSqrt  SaturateOnIntegerOverflow=on
  rad2deg : Gain  Gain=180/pi
  Th1 [%] : Outport
  Th2 [%] : Outport  Port=2
  Th3 [%] : Outport  Port=3
  Th4 [%] : Outport  Port=4
  Alpha1 [deg] : Outport  Port=5
  Alpha2 [deg] : Outport  Port=6
  Alpha3 [deg] : Outport  Port=7
  Alpha4 [deg] : Outport  Port=8
  wires:
  Saturation6/1 -> Alpha3 [deg]/1
  Demux2/1 -> Saturation4/1
  Demux2/3 -> Saturation6/1
  Sqrt1/1 -> Bias1/1
  Bias1/1 -> Gain3/1
  Demux2/2 -> Saturation5/1
  Demux2/4 -> Saturation7/1
  Saturation4/1 -> Alpha1 [deg]/1
  Saturation5/1 -> Alpha2 [deg]/1
  Saturation7/1 -> Alpha4 [deg]/1
  Fx/1 -> Mux/1
  Fy/1 -> Mux/2
  T/1 -> Mux/3
  L/1 -> Mux/4
  M/1 -> Mux/5
  N/1 -> Mux/6
  Selector/1 -> Sqrt1/1
  Selector1/1 -> rad2deg/1
  rad2deg/1 -> Demux2/1
  Gain2/1 -> Selector1/1, Selector/1
  Mux/1 -> Gain2/1
  Demux1/3 -> Saturation3/1
  Demux1/2 -> Saturation2/1
  Demux1/4 -> Saturation8/1
  Demux1/1 -> Saturation1/1
  Saturation1/1 -> Th1 [%]/1
  Saturation2/1 -> Th2 [%]/1
  Saturation3/1 -> Th3 [%]/1
  Saturation8/1 -> Th4 [%]/1
  Gain3/1 -> Demux1/1  "Th [%]"

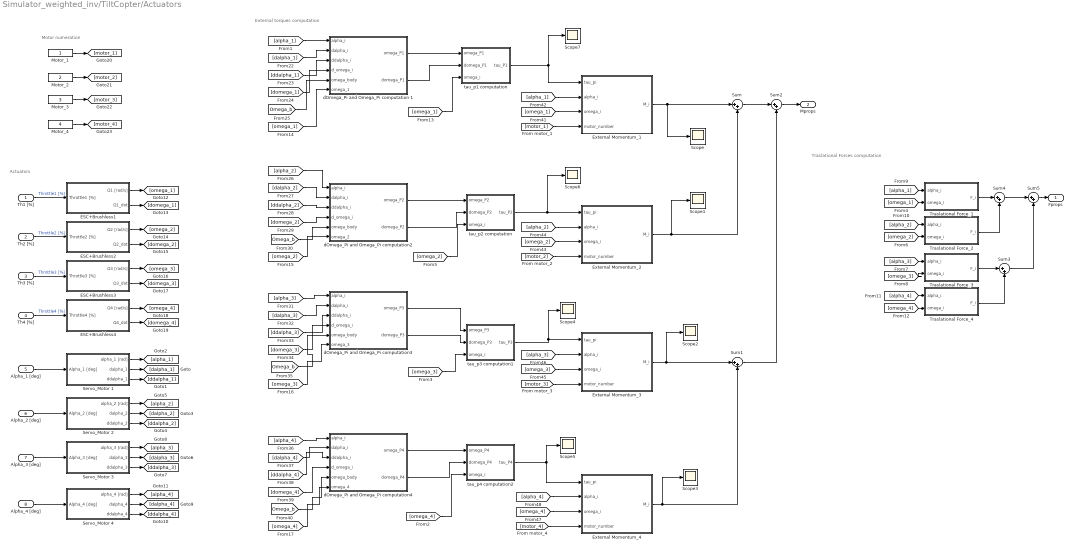
== system Simulator_weighted_inv/TiltCopter/Actuators ==
  note: Actuators
  note: Motor numeration
  note: External torques computation
  note: Traslational Forces computation
  Th1 [%] : Inport
  Th2 [%] : Inport  Port=2
  Th3 [%] : Inport  Port=3
  Th4 [%] : Inport  Port=4
  Alpha_1 [deg] : Inport  Port=5
  Alpha_2 [deg] : Inport  Port=6
  Alpha_3 [deg] : Inport  Port=7
  Alpha_4 [deg] : Inport  Port=8
  ESC+Brushless1 : Subsystem
  ESC+Brushless2 : Subsystem
  ESC+Brushless3 : Subsystem
  ESC+Brushless4 : Subsystem
  External Momentum_1 : Subsystem
  External Momentum_2 : Subsystem
  External Momentum_3 : Subsystem
  External Momentum_4 : Subsystem
  Motor_1 : Constant
  Motor_2 : Constant  Value=2
  Motor_3 : Constant  Value=3
  Motor_4 : Constant  Value=4
  Scope{,1..7} (8 alike) : Scope
  Servo_Motor 1 : Subsystem
  Servo_Motor 2 : Subsystem
  Servo_Motor 3 : Subsystem
  Servo_Motor 4 : Subsystem
  Sum{,1..5} (6 alike) : Sum  Inputs=|++
  Traslational Force_1 : Subsystem
  Traslational Force_2 : Subsystem
  Traslational Force_3 : Subsystem
  Traslational Force_4 : Subsystem
  dOmega_Pi and Omega_Pi computation 1 : Subsystem
  dOmega_Pi and Omega_Pi computation2 : Subsystem
  dOmega_Pi and Omega_Pi computation3 : Subsystem
  dOmega_Pi and Omega_Pi computation4 : Subsystem
  tau_p1 computation : Subsystem
  tau_p2 computation : Subsystem
  tau_p3 computation1 : Subsystem
  tau_p4 computation2 : Subsystem
  Fprops : Outport
  Mprops : Outport  Port=2
  wires:
  Th1 [%]/1 -> ESC+Brushless1/1(Throttle1 [%])  "Throttle1 [%]"
  Th2 [%]/1 -> ESC+Brushless2/1(Throttle2 [%])  "Throttle2 [%]"
  Th4 [%]/1 -> ESC+Brushless4/1(Throttle4 [%])  "Throttle4 [%]"
  Th3 [%]/1 -> ESC+Brushless3/1(Throttle3 [%])  "Throttle3 [%]"
  Alpha_1 [deg]/1 -> Servo_Motor 1/1(Alpha_1 [deg])
  Servo_Motor 1/2(dalpha_1) -> [dalpha_1]
  Servo_Motor 1/3(ddalpha_1) -> [ddalpha_1]
  Servo_Motor 3/1(alpha_3 [rad]) -> [alpha_3]
  Servo_Motor 3/3(ddalpha_3) -> [ddalpha_3]
  Servo_Motor 3/2(dalpha_3) -> [dalpha_3]
  Servo_Motor 2/3(ddalpha_2) -> [ddalpha_2]
  Servo_Motor 2/2(dalpha_2) -> [dalpha_2]
  Servo_Motor 2/1(alpha_2 [rad]) -> [alpha_2]
  Servo_Motor 1/1(alpha_1 [rad]) -> [alpha_1]
  Servo_Motor 4/1(alpha_4 [rad]) -> [alpha_4]
  Servo_Motor 4/2(dalpha_4) -> [dalpha_4]
  Servo_Motor 4/3(ddalpha_4) -> [ddalpha_4]
  ESC+Brushless1/1(Ω1 [rad/s]) -> [omega_1]
  ESC+Brushless1/2(Ω1_dot) -> [domega_1]
  ESC+Brushless2/1(Ω2 [rad/s]) -> [omega_2]
  ESC+Brushless3/1(Ω3 [rad/s]) -> [omega_3]
  ESC+Brushless3/2(Ω3_dot) -> [domega_3]
  ESC+Brushless4/1(Ω4 [rad/s]) -> [omega_4]
  ESC+Brushless4/2("Ω4_dot ") -> [domega_4]
  [alpha_1] -> dOmega_Pi and Omega_Pi computation 1/1(alpha_i)
  [dalpha_1] -> dOmega_Pi and Omega_Pi computation 1/2(dalpha_i)
  [ddalpha_1] -> dOmega_Pi and Omega_Pi computation 1/3(ddalpha_i)
  [domega_1] -> dOmega_Pi and Omega_Pi computation 1/4(d_omega_i)
  [Omega_b] -> dOmega_Pi and Omega_Pi computation 1/5(omega_body)
  [alpha_2] -> dOmega_Pi and Omega_Pi computation2/1(alpha_i)
  [dalpha_2] -> dOmega_Pi and Omega_Pi computation2/2(dalpha_i)
  [ddalpha_2] -> dOmega_Pi and Omega_Pi computation2/3(ddalpha_i)
  [domega_2] -> dOmega_Pi and Omega_Pi computation2/4(d_omega_i)
  [Omega_b] -> dOmega_Pi and Omega_Pi computation2/5(omega_body)
  [alpha_3] -> dOmega_Pi and Omega_Pi computation3/1(alpha_i)
  [dalpha_3] -> dOmega_Pi and Omega_Pi computation3/2(dalpha_i)
  [ddalpha_3] -> dOmega_Pi and Omega_Pi computation3/3(ddalpha_i)
  [domega_3] -> dOmega_Pi and Omega_Pi computation3/4(d_omega_i)
  [Omega_b] -> dOmega_Pi and Omega_Pi computation3/5(omega_body)
  [alpha_4] -> dOmega_Pi and Omega_Pi computation4/1(alpha_i)
  [dalpha_4] -> dOmega_Pi and Omega_Pi computation4/2(dalpha_i)
  [ddalpha_4] -> dOmega_Pi and Omega_Pi computation4/3(ddalpha_i)
  [domega_4] -> dOmega_Pi and Omega_Pi computation4/4(d_omega_i)
  [Omega_b] -> dOmega_Pi and Omega_Pi computation4/5(omega_body)
  dOmega_Pi and Omega_Pi computation 1/1(omega_P1) -> tau_p1 computation/1(omega_P1)
  dOmega_Pi and Omega_Pi computation 1/2(domega_P1) -> tau_p1 computation/2(domega_P1)
  dOmega_Pi and Omega_Pi computation2/1(omega_P2) -> tau_p2 computation/1(omega_P2)
  dOmega_Pi and Omega_Pi computation2/2(domega_P2) -> tau_p2 computation/2(domega_P2)
  dOmega_Pi and Omega_Pi computation3/1(omega_P3) -> tau_p3 computation1/1(omega_P3)
  dOmega_Pi and Omega_Pi computation3/2(domega_P3) -> tau_p3 computation1/2(domega_P3)
  dOmega_Pi and Omega_Pi computation4/1(omega_P4) -> tau_p4 computation2/1(omega_P4)
  dOmega_Pi and Omega_Pi computation4/2(domega_P4) -> tau_p4 computation2/2(domega_P4)
  tau_p1 computation/1(tau_P1) -> External Momentum_1/1(tau_pi), Scope7/1
  [alpha_1] -> External Momentum_1/2(alpha_i)
  [omega_1] -> External Momentum_1/3(omega_i)
  tau_p2 computation/1(tau_P2) -> Scope6/1, External Momentum_2/1(tau_pi)
  [alpha_2] -> External Momentum_2/2(alpha_i)
  [omega_2] -> External Momentum_2/3(omega_i)
  [motor_2] -> External Momentum_2/4(motor_number)
  tau_p3 computation1/1(tau_P3) -> Scope4/1, External Momentum_3/1(tau_pi)
  [alpha_3] -> External Momentum_3/2(alpha_i)
  [omega_3] -> External Momentum_3/3(omega_i)
  [motor_3] -> External Momentum_3/4(motor_number)
  [alpha_4] -> External Momentum_4/2(alpha_i)
  [omega_4] -> External Momentum_4/3(omega_i)
  [motor_4] -> External Momentum_4/4(motor_number)
  tau_p4 computation2/1(tau_P4) -> Scope5/1, External Momentum_4/1(tau_pi)
  External Momentum_1/1(M_i) -> Scope/1, Sum/1
  External Momentum_3/1(M_i) -> Scope2/1, Sum1/1
  External Momentum_4/1(M_i) -> Scope3/1, Sum1/2
  Sum/1 -> Sum2/1
  Sum2/1 -> Mprops/1
  [omega_2] -> Traslational Force_2/2(omega_i)
  [alpha_1] -> Traslational Force_1/1(alpha_i)
  [omega_1] -> Traslational Force_1/2(omega_i)
  [alpha_2] -> Traslational Force_2/1(alpha_i)
  Motor_1/1 -> [motor_1]
  Motor_2/1 -> [motor_2]
  Motor_3/1 -> [motor_3]
  Motor_4/1 -> [motor_4]
  [omega_3] -> Traslational Force_3/2(omega_i)
  [alpha_3] -> Traslational Force_3/1(alpha_i)
  [omega_4] -> Traslational Force_4/2(omega_i)
  [alpha_4] -> Traslational Force_4/1(alpha_i)
  Traslational Force_3/1(F_i) -> Sum3/1
  Traslational Force_4/1(F_i) -> Sum3/2
  Traslational Force_1/1(F_i) -> Sum4/1
  Traslational Force_2/1(F_i) -> Sum4/2
  Sum4/1 -> Sum5/1
  Sum3/1 -> Sum5/2
  Sum5/1 -> Fprops/1
  [omega_4] -> tau_p4 computation2/3(omega_i)
  [omega_3] -> tau_p3 computation1/3(omega_i)
  [omega_2] -> tau_p2 computation/3(omega_i)
  [omega_1] -> tau_p1 computation/3(omega_i)
  Sum1/1 -> Sum2/2
  External Momentum_2/1(M_i) -> Scope1/1, Sum/2
  [omega_1] -> dOmega_Pi and Omega_Pi computation 1/6(omega_1)
  [omega_2] -> dOmega_Pi and Omega_Pi computation2/6(omega_2)
  [omega_3] -> dOmega_Pi and Omega_Pi computation3/6(omega_3)
  [omega_4] -> dOmega_Pi and Omega_Pi computation4/6(omega_4)
  ESC+Brushless2/2(Ω2_dot) -> [domega_2]
  Alpha_2 [deg]/1 -> Servo_Motor 2/1(Alpha_2 [deg])
  Alpha_3 [deg]/1 -> Servo_Motor 3/1(Alpha_3 [deg])
  Alpha_4 [deg]/1 -> Servo_Motor 4/1(Alpha_4 [deg])
  [motor_1] -> External Momentum_1/4(motor_number)

== system Simulator_weighted_inv/TiltCopter/Actuators/ESC+Brushless1 ==
  Throttle1 [%] : Inport
  Subsystem : Subsystem
  Ω1 [rad/s] : Outport
  Ω1_dot : Outport  Port=2
  wires:
  Subsystem/1(omega_i) -> Ω1 [rad/s]/1
  Subsystem/2(domega_i) -> Ω1_dot/1
  Throttle1 [%]/1 -> Subsystem/1(Throttle [%])

== system Simulator_weighted_inv/TiltCopter/Actuators/ESC+Brushless2 ==
  Throttle2 [%] : Inport
  Subsystem : Subsystem
  Ω2 [rad/s] : Outport
  Ω2_dot : Outport  Port=2
  wires:
  Throttle2 [%]/1 -> Subsystem/1(Throttle [%])
  Subsystem/1(omega_i) -> Ω2 [rad/s]/1
  Subsystem/2(domega_i) -> Ω2_dot/1

== system Simulator_weighted_inv/TiltCopter/Actuators/ESC+Brushless3 ==
  Throttle3 [%] : Inport
  Subsystem : Subsystem
  Ω3 [rad/s] : Outport
  Ω3_dot : Outport  Port=2
  wires:
  Throttle3 [%]/1 -> Subsystem/1(Throttle [%])
  Subsystem/2(domega_i) -> Ω3_dot/1
  Subsystem/1(omega_i) -> Ω3 [rad/s]/1

== system Simulator_weighted_inv/TiltCopter/Actuators/ESC+Brushless4 ==
  Throttle4 [%] : Inport
  Subsystem : Subsystem
  Ω4 [rad/s] : Outport
  "Ω4_dot " : Outport  Port=2
  wires:
  Throttle4 [%]/1 -> Subsystem/1(Throttle [%])
  Subsystem/2(domega_i) -> "Ω4_dot "/1
  Subsystem/1(omega_i) -> Ω4 [rad/s]/1

== system Simulator_weighted_inv/TiltCopter/Actuators/External Momentum_1 ==
  tau_pi : Inport
  alpha_i : Inport  Port=2
  omega_i : Inport  Port=3
  motor_number : Inport  Port=4
  3x3 Cross Product : aerolibutil/3x3 Cross Product
  O_BPi : MATLAB Function  TreatAsAtomicUnit=on
  Product : Product  Multiplication=Matrix(*)
  Product1 : Product  Multiplication=Matrix(*)
  R_BP1 : MATLAB Function  TreatAsAtomicUnit=on
  Sum : Sum  Inputs=-+|
  Thrust computation : Subsystem
  M_i : Outport
  wires:
  Sum/1 -> M_i/1
  R_BP1/1(Rotation_matrix) -> Product1/1, Product/1
  alpha_i/1 -> R_BP1/1(alpha_1)
  Product/1 -> 3x3 Cross Product/2
  tau_pi/1 -> Product1/2
  motor_number/1 -> O_BPi/1(motor_number)
  omega_i/1 -> Thrust computation/1(omega_i)
  Thrust computation/1(Vector_Thrust_i) -> Product/2
  3x3 Cross Product/1 -> Sum/2
  Product1/1 -> Sum/1
  O_BPi/1(Origin_Rotation) -> 3x3 Cross Product/1

== system Simulator_weighted_inv/TiltCopter/Actuators/External Momentum_2 ==
  tau_pi : Inport
  alpha_i : Inport  Port=2
  omega_i : Inport  Port=3
  motor_number : Inport  Port=4
  3x3 Cross Product : aerolibutil/3x3 Cross Product
  O_BPi : MATLAB Function  TreatAsAtomicUnit=on
  Product : Product  Multiplication=Matrix(*)
  Product1 : Product  Multiplication=Matrix(*)
  R_BP2 : MATLAB Function  TreatAsAtomicUnit=on
  Sum : Sum  Inputs=-+|
  Thrust computation : Subsystem
  M_i : Outport
  wires:
  Sum/1 -> M_i/1
  R_BP2/1(Rotation_matrix) -> Product1/1, Product/1
  alpha_i/1 -> R_BP2/1(alpha_2)
  Product/1 -> 3x3 Cross Product/2
  tau_pi/1 -> Product1/2
  motor_number/1 -> O_BPi/1(motor_number)
  omega_i/1 -> Thrust computation/1(omega_i)
  Thrust computation/1(Vector_Thrust_i) -> Product/2
  3x3 Cross Product/1 -> Sum/2
  Product1/1 -> Sum/1
  O_BPi/1(Origin_Rotation) -> 3x3 Cross Product/1

== system Simulator_weighted_inv/TiltCopter/Actuators/External Momentum_3 ==
  tau_pi : Inport
  alpha_i : Inport  Port=2
  omega_i : Inport  Port=3
  motor_number : Inport  Port=4
  3x3 Cross Product : aerolibutil/3x3 Cross Product
  O_BPi : MATLAB Function  TreatAsAtomicUnit=on
  Product : Product  Multiplication=Matrix(*)
  Product1 : Product  Multiplication=Matrix(*)
  R_BP3 : MATLAB Function  TreatAsAtomicUnit=on
  Sum : Sum  Inputs=-+|
  Thrust computation : Subsystem
  M_i : Outport
  wires:
  Sum/1 -> M_i/1
  R_BP3/1(Rotation_matrix) -> Product1/1, Product/1
  alpha_i/1 -> R_BP3/1(alpha_3)
  Product/1 -> 3x3 Cross Product/2
  tau_pi/1 -> Product1/2
  motor_number/1 -> O_BPi/1(motor_number)
  omega_i/1 -> Thrust computation/1(omega_i)
  Thrust computation/1(Vector_Thrust_i) -> Product/2
  3x3 Cross Product/1 -> Sum/2
  Product1/1 -> Sum/1
  O_BPi/1(Origin_Rotation) -> 3x3 Cross Product/1

== system Simulator_weighted_inv/TiltCopter/Actuators/External Momentum_4 ==
  tau_pi : Inport
  alpha_i : Inport  Port=2
  omega_i : Inport  Port=3
  motor_number : Inport  Port=4
  3x3 Cross Product : aerolibutil/3x3 Cross Product
  O_BPi : MATLAB Function  TreatAsAtomicUnit=on
  Product : Product  Multiplication=Matrix(*)
  Product1 : Product  Multiplication=Matrix(*)
  R_BP4 : MATLAB Function  TreatAsAtomicUnit=on
  Sum : Sum  Inputs=-+|
  Thrust computation : Subsystem
  M_i : Outport
  wires:
  Sum/1 -> M_i/1
  R_BP4/1(Rotation_matrix) -> Product1/1, Product/1
  alpha_i/1 -> R_BP4/1(alpha_4)
  Product/1 -> 3x3 Cross Product/2
  tau_pi/1 -> Product1/2
  motor_number/1 -> O_BPi/1(motor_number)
  omega_i/1 -> Thrust computation/1(omega_i)
  Thrust computation/1(Vector_Thrust_i) -> Product/2
  3x3 Cross Product/1 -> Sum/2
  Product1/1 -> Sum/1
  O_BPi/1(Origin_Rotation) -> 3x3 Cross Product/1

== system Simulator_weighted_inv/TiltCopter/Actuators/Servo_Motor 1 ==
  Alpha_1 [deg] : Inport
  Demux : Demux  Outputs=3
  State-Space : StateSpace  A=A_Servo  B=B_Servo  C=C_Servo  D=[0 0 0]'  X0=[0 0 0 ]  ContinuousStateAttributes=['alpha' 'dalpha' 'ddalpha']
  deg2rad : Gain  Gain=pi/180
  alpha_1 [rad] : Outport
  dalpha_1 : Outport  Port=2
  ddalpha_1 : Outport  Port=3
  wires:
  deg2rad/1 -> State-Space/1
  Alpha_1 [deg]/1 -> deg2rad/1
  State-Space/1 -> Demux/1
  Demux/1 -> alpha_1 [rad]/1
  Demux/2 -> dalpha_1/1
  Demux/3 -> ddalpha_1/1
